simulink model "ArmA"  (R2017a)
settings: Solver=VariableStepAuto  StartTime=0.0  StopTime=10.0  RelTol=1e-3
undefined symbols (not defined in the file): base, link1, link2
libraries: mblibv1 x10
settings Model: Creator=Smile  LastModifiedBy=Smile
settings SimMechanicsCC: VisOnUpdateDiagram=on  VisDuringSimulation=on

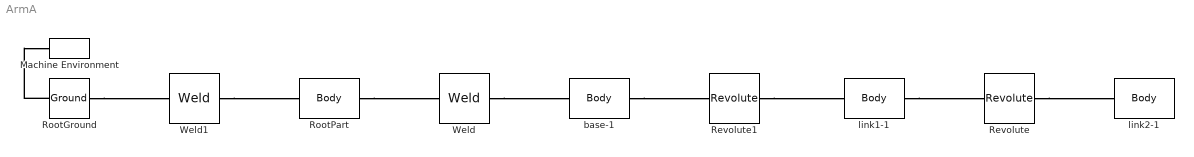
== system ArmA ==
  Machine Environment : mblibv1/Bodies/Machine Environment  PortType=env  PhysicalDomain=Mechanical  DialogTemplateClass=MECH.MachineEnvironment  SyncWhenCopied=off  Gravity=[0 -9.81 0]  GravityUnits=m/s^2  GravityAsSignal=off  Dimensionality=Auto-detect  AnalysisType=Forward dynamics  LinearAssemblyTolerance=1e-3  LinearAssemblyToleranceUnits=m  AngularAssemblyTolerance=1e-3  AngularAssemblyToleranceUnits=rad  ConstraintSolverType=Stabilizing  ConstraintRelTolerance=1e-4  ConstraintAbsTolerance=1e-4  UseRobustSingularityHandling=off  RedundancyAnalysisToleranceType=Automatically select tolerance  RedundancyAnalysisTolerance=1e-14  StatePerturbationType=Fixed  PerturbationSize=1e-5  VisualizeMachine=on  BodyVisualizationType=Use model default body geometries  BodyColorSelMode=Use model default  DefaultBodyColor=[1 0 0]
      settings: SourceProductName=Simscape Multibody  SourceProductBaseCode=MS
  Revolute : mblibv1/Joints/Revolute  LConnTagsString=__newl0  RConnTagsString=__newr0  UpdateFromCAD=on  PMImportedID=link1-1:-:link2-1  NumSAPorts=0  CutJoint=off  MarkAsCut=off  Primitives=prismatic  PrimitiveProps=R1$WORLD$[-1,0,0]$revolute  DialogClass=JointBlock  R1Axis=[-1,0,0]
      settings: SourceProductName=Simscape Multibody  SourceProductBaseCode=MS
  Revolute1 : mblibv1/Joints/Revolute  LConnTagsString=__newl0  RConnTagsString=__newr0  UpdateFromCAD=on  PMImportedID=base-1:-:link1-1  NumSAPorts=0  CutJoint=off  MarkAsCut=off  Primitives=prismatic  PrimitiveProps=R1$WORLD$[-1,0,0]$revolute  DialogClass=JointBlock  R1Axis=[-1,0,0]
      settings: SourceProductName=Simscape Multibody  SourceProductBaseCode=MS
  RootGround : mblibv1/Bodies/Ground  UpdateFromCAD=on  PMImportedID=RootGround  LeftPortType=env  RightPortType=workingframe  PhysicalDomain=Mechanical  DialogClass=GroundBlock  CoordPosition=[0.0498083,0.139315,0.175583]  CoordPositionUnits=m  StateVectorMgrId=-1  MachineId=[0 0]  ShowEnvPort=on  ParameterChecksum=[0 0 0 0]  TopologyChecksum=[0 0 0 0]
      settings: SourceProductName=Simscape Multibody  SourceProductBaseCode=MS
  RootPart : mblibv1/Bodies/Body  LConnTagsString=CS3  RConnTagsString=CS2  UpdateFromCAD=on  PMImportedID=ArmA/RootPart  DialogClass=MechanicalBodyBlock  Mass=0  MassUnits=kg  InertiaUnits=kg*m^2  Inertia=[0,0,0;0,0,0;0,0,0]  Shape=Cylinder  ShapeDims=[1 1]  ShapeUnits=m  ShapeUse=false  Density=1  DensityUnits=kg/m^3  DensityUse=false  GraphicsMode=MACHINE_DEFAULT  BodyColorSelMode=MACHINE_DEFAULT  BodyColor=[1;0;0]  AttachedToCS=CS1  CG=Right$CG$[0.0498083 0.139315 0.175583]$WORLD$WORLD$m$[1 0 0;0 1 0;0 0 1]$3x3 Transform$rad$WORLD$false$ArmA/RootPart::CG(AUTOGEN)  WorkingFrames=Right$CS1$[0 0 0]$WORLD$WORLD$m$[1 0 0;0 1 0;0 0 1]$3x3 Transform$rad$WORLD$false$ArmA/RootPart::CS1(AUTOGEN)#Right$CS2$[0.0528389 0.105422 0.184564]$WORLD$WORLD$m$[1 0 0;0 1 0;0 0 1]$3x3 Transform$rad$WORLD$true$ArmA/RootPart:-:base-1::ArmA/RootPart(AUTOGEN)#Left$CS3$[0.0498083 0.139315 0.175583]$WORLD$WORLD$m$[1 0 0;0 1 0;0 0 1]$3x3 Transform$rad$WORLD$true$ArmA/RootPart:-:RootGround::ArmA/RootPart(AUTOGEN)  CGPos=[0.0498083 0.139315 0.175583]  CGRot=[1 0 0;0 1 0;0 0 1]  CS0Pos=[]  CS0Rot=[]  CS1Pos=[0 0 0]  CS1Rot=[1 0 0;0 1 0;0 0 1]  CS2Pos=[0.0528389 0.105422 0.184564]  CS2Rot=[1 0 0;0 1 0;0 0 1]  CS3Pos=[0.0498083 0.139315 0.175583]  CS3Rot=[1 0 0;0 1 0;0 0 1]  CS4Pos=[]  CS4Rot=[]  CS5Pos=[]  CS5Rot=[]  CS6Pos=[]  CS6Rot=[]  CS7Pos=[]  CS7Rot=[]  CS8Pos=[]  CS8Rot=[]  CS9Pos=[]  CS9Rot=[]  CS10Pos=[]  CS10Rot=[]  CS11Pos=[]  CS11Rot=[]  CS12Pos=[]  CS12Rot=[]  CS13Pos=[]  CS13Rot=[]  CS14Pos=[]  CS14Rot=[]  CS15Pos=[]  CS15Rot=[]  CS16Pos=[]  CS16Rot=[]  CS17Pos=[]  CS17Rot=[]  CS18Pos=[]  CS18Rot=[]  CS19Pos=[]  CS19Rot=[]  CS20Pos=[]  CS20Rot=[]
      settings: SourceProductName=Simscape Multibody  SourceProductBaseCode=MS
  Weld : mblibv1/Joints/Weld  LConnTagsString=__newl0  RConnTagsString=__newr0  UpdateFromCAD=on  PMImportedID=ArmA/RootPart:-:base-1  NumSAPorts=0  CutJoint=off  MarkAsCut=off  Primitives=weld  PrimitiveProps=W$WORLD$[0.57735,0.57735,0.57735]$weld  DialogClass=JointBlock  WAxis=[0.57735,0.57735,0.57735]
      settings: SourceProductName=Simscape Multibody  SourceProductBaseCode=MS
  Weld1 : mblibv1/Joints/Weld  LConnTagsString=__newl0  RConnTagsString=__newr0  UpdateFromCAD=on  PMImportedID=ArmA/RootPart:-:RootGround  NumSAPorts=0  CutJoint=off  MarkAsCut=off  Primitives=weld  PrimitiveProps=W$WORLD$[0.57735,0.57735,0.57735]$weld  DialogClass=JointBlock  WAxis=[0.57735,0.57735,0.57735]
      settings: SourceProductName=Simscape Multibody  SourceProductBaseCode=MS
  base-1 : mblibv1/Bodies/Body  LConnTagsString=CS2  RConnTagsString=CS3  UpdateFromCAD=on  PMImportedID=base-1  DialogClass=MechanicalBodyBlock  Mass=0.00014284  MassUnits=kg  InertiaUnits=kg*m^2  Inertia=[4.29076e-07,0,0;0,2.79086e-07,0;0,0,6.85126e-07]  Shape=Cylinder  ShapeDims=[1 1]  ShapeUnits=m  ShapeUse=false  Density=1  DensityUnits=kg/m^3  DensityUse=false  GraphicsMode=GFXFILE  GraphicsFileName=ArmA - base-1.STL  BodyColorSelMode=COLORPALETTE  BodyColor=[0.792157;0.819608;0.933333]  AttachedToCS=CS1  CG=Right$CG$[0.0528389 0.105422 0.184564]$WORLD$WORLD$m$[1 0 0;0 1 0;0 0 1]$3x3 Transform$rad$WORLD$false$base-1::CG(AUTOGEN)  WorkingFrames=Right$CS1$[-0.0159917 0.016192 0.020438]$WORLD$WORLD$m$[1 0 0;0 1 0;0 0 1]$3x3 Transform$rad$WORLD$false$base-1::CS1(AUTOGEN)#Left$CS2$[0.0528389 0.105422 0.184564]$WORLD$WORLD$m$[1 0 0;0 1 0;0 0 1]$3x3 Transform$rad$WORLD$true$ArmA/RootPart:-:base-1::base-1(AUTOGEN)#Right$CS3$[0.0668389 0.105422 0.164315]$WORLD$WORLD$m$[1 0 0;0 1 0;0 0 1]$3x3 Transform$rad$WORLD$true$base-1:-:link1-1::base-1(AUTOGEN)  CGPos=[0.0528389 0.105422 0.184564]  CGRot=[1 0 0;0 1 0;0 0 1]  CS0Pos=[]  CS0Rot=[]  CS1Pos=[-0.0159917 0.016192 0.020438]  CS1Rot=[1 0 0;0 1 0;0 0 1]  CS2Pos=[0.0528389 0.105422 0.184564]  CS2Rot=[1 0 0;0 1 0;0 0 1]  CS3Pos=[0.0668389 0.105422 0.164315]  CS3Rot=[1 0 0;0 1 0;0 0 1]  CS4Pos=[]  CS4Rot=[]  CS5Pos=[]  CS5Rot=[]  CS6Pos=[]  CS6Rot=[]  CS7Pos=[]  CS7Rot=[]  CS8Pos=[]  CS8Rot=[]  CS9Pos=[]  CS9Rot=[]  CS10Pos=[]  CS10Rot=[]  CS11Pos=[]  CS11Rot=[]  CS12Pos=[]  CS12Rot=[]  CS13Pos=[]  CS13Rot=[]  CS14Pos=[]  CS14Rot=[]  CS15Pos=[]  CS15Rot=[]  CS16Pos=[]  CS16Rot=[]  CS17Pos=[]  CS17Rot=[]  CS18Pos=[]  CS18Rot=[]  CS19Pos=[]  CS19Rot=[]  CS20Pos=[]  CS20Rot=[]
      settings: SourceProductName=Simscape Multibody  SourceProductBaseCode=MS
  link1-1 : mblibv1/Bodies/Body  LConnTagsString=CS3  RConnTagsString=CS2  UpdateFromCAD=on  PMImportedID=link1-1  DialogClass=MechanicalBodyBlock  Mass=5.18149e-05  MassUnits=kg  InertiaUnits=kg*m^2  Inertia=[8.65344e-08,-1.85431e-10,4.69279e-13;-1.85431e-10,7.42955e-09,4.60196e-10;4.69279e-13,4.60196e-10,8.43164e-08]  Shape=Cylinder  ShapeDims=[1 1]  ShapeUnits=m  ShapeUse=false  Density=1  DensityUnits=kg/m^3  DensityUse=false  GraphicsMode=GFXFILE  GraphicsFileName=ArmA - link1-1.STL  BodyColorSelMode=COLORPALETTE  BodyColor=[0.792157;0.819608;0.933333]  AttachedToCS=CS1  CG=Right$CG$[0.0528893 0.139602 0.163744]$WORLD$WORLD$m$[1 0 0;0 0.999704 0.024314;0 -0.024314 0.999704]$3x3 Transform$rad$WORLD$false$link1-1::CG(AUTOGEN)  WorkingFrames=Right$CS1$[-0.0159917 0.0127202 0.02265]$WORLD$WORLD$m$[1 0 0;0 0.999704 0.024314;0 -0.024314 0.999704]$3x3 Transform$rad$WORLD$false$link1-1::CS1(AUTOGEN)#Right$CS2$[0.0428389 0.205392 0.161884]$WORLD$WORLD$m$[1 0 0;0 1 0;0 0 1]$3x3 Transform$rad$WORLD$true$link1-1:-:link2-1::link1-1(AUTOGEN)#Left$CS3$[0.0668389 0.105422 0.164315]$WORLD$WORLD$m$[1 0 0;0 1 0;0 0 1]$3x3 Transform$rad$WORLD$true$base-1:-:link1-1::link1-1(AUTOGEN)  CGPos=[0.0528893 0.139602 0.163744]  CGRot=[1 0 0;0 0.999704 0.024314;0 -0.024314 0.999704]  CS0Pos=[]  CS0Rot=[]  CS1Pos=[-0.0159917 0.0127202 0.02265]  CS1Rot=[1 0 0;0 0.999704 0.024314;0 -0.024314 0.999704]  CS2Pos=[0.0428389 0.205392 0.161884]  CS2Rot=[1 0 0;0 1 0;0 0 1]  CS3Pos=[0.0668389 0.105422 0.164315]  CS3Rot=[1 0 0;0 1 0;0 0 1]  CS4Pos=[]  CS4Rot=[]  CS5Pos=[]  CS5Rot=[]  CS6Pos=[]  CS6Rot=[]  CS7Pos=[]  CS7Rot=[]  CS8Pos=[]  CS8Rot=[]  CS9Pos=[]  CS9Rot=[]  CS10Pos=[]  CS10Rot=[]  CS11Pos=[]  CS11Rot=[]  CS12Pos=[]  CS12Rot=[]  CS13Pos=[]  CS13Rot=[]  CS14Pos=[]  CS14Rot=[]  CS15Pos=[]  CS15Rot=[]  CS16Pos=[]  CS16Rot=[]  CS17Pos=[]  CS17Rot=[]  CS18Pos=[]  CS18Rot=[]  CS19Pos=[]  CS19Rot=[]  CS20Pos=[]  CS20Rot=[]
      settings: SourceProductName=Simscape Multibody  SourceProductBaseCode=MS
  link2-1 : mblibv1/Bodies/Body  LConnTagsString=CS2  UpdateFromCAD=on  PMImportedID=link2-1  DialogClass=MechanicalBodyBlock  Mass=5.02929e-05  MassUnits=kg  InertiaUnits=kg*m^2  Inertia=[6.85166e-08,-9.0051e-10,1.17293e-11;-9.0051e-10,7.99347e-09,-4.09433e-10;1.17293e-11,-4.09433e-10,6.76463e-08]  Shape=Cylinder  ShapeDims=[1 1]  ShapeUnits=m  ShapeUse=false  Density=1  DensityUnits=kg/m^3  DensityUse=false  GraphicsMode=GFXFILE  GraphicsFileName=ArmA - link2-1.STL  BodyColorSelMode=COLORPALETTE  BodyColor=[0.792157;0.819608;0.933333]  AttachedToCS=CS1  CG=Right$CG$[0.0380268 0.235283 0.162273]$WORLD$WORLD$m$[1 0 0;0 0.999755 -0.0221121;0 0.0221121 0.999755]$3x3 Transform$rad$WORLD$false$link2-1::CG(AUTOGEN)  WorkingFrames=Right$CS1$[-0.0159917 0.0193902 0.0138575]$WORLD$WORLD$m$[1 0 0;0 0.999755 -0.0221121;0 0.0221121 0.999755]$3x3 Transform$rad$WORLD$false$link2-1::CS1(AUTOGEN)#Left$CS2$[0.0428389 0.205392 0.161884]$WORLD$WORLD$m$[1 0 0;0 1 0;0 0 1]$3x3 Transform$rad$WORLD$true$link1-1:-:link2-1::link2-1(AUTOGEN)  CGPos=[0.0380268 0.235283 0.162273]  CGRot=[1 0 0;0 0.999755 -0.0221121;0 0.0221121 0.999755]  CS0Pos=[]  CS0Rot=[]  CS1Pos=[-0.0159917 0.0193902 0.0138575]  CS1Rot=[1 0 0;0 0.999755 -0.0221121;0 0.0221121 0.999755]  CS2Pos=[0.0428389 0.205392 0.161884]  CS2Rot=[1 0 0;0 1 0;0 0 1]  CS3Pos=[]  CS3Rot=[]  CS4Pos=[]  CS4Rot=[]  CS5Pos=[]  CS5Rot=[]  CS6Pos=[]  CS6Rot=[]  CS7Pos=[]  CS7Rot=[]  CS8Pos=[]  CS8Rot=[]  CS9Pos=[]  CS9Rot=[]  CS10Pos=[]  CS10Rot=[]  CS11Pos=[]  CS11Rot=[]  CS12Pos=[]  CS12Rot=[]  CS13Pos=[]  CS13Rot=[]  CS14Pos=[]  CS14Rot=[]  CS15Pos=[]  CS15Rot=[]  CS16Pos=[]  CS16Rot=[]  CS17Pos=[]  CS17Rot=[]  CS18Pos=[]  CS18Rot=[]  CS19Pos=[]  CS19Rot=[]  CS20Pos=[]  CS20Rot=[]
      settings: SourceProductName=Simscape Multibody  SourceProductBaseCode=MS
  connections:
  RootPart/RConn1 -- Weld/LConn1
  Weld/RConn1 -- base-1/LConn1
  link1-1/RConn1 -- Revolute/LConn1
  Revolute/RConn1 -- link2-1/LConn1
  base-1/RConn1 -- Revolute1/LConn1
  Revolute1/RConn1 -- link1-1/LConn1
  RootGround/RConn1 -- Weld1/LConn1
  Weld1/RConn1 -- RootPart/LConn1
  RootGround/LConn1 -- Machine Environment/RConn1
